simulink model "greenhouse_simulink_part3_pid"  (R2023b)
settings: Solver=VariableStepAuto  StartTime=0.0  StopTime=60*60*24  RelTol=1e-3
undefined symbols (not defined in the file or in its folder): Ca, km1_m2, km1e, km2e, p, t0, thermal_pump, Ts
libraries: slpidlib x2
settings Model: Creator=bianc  LastModifiedBy=bianc
settings OptimizationCC: ReuseModelBlockBuffer=off

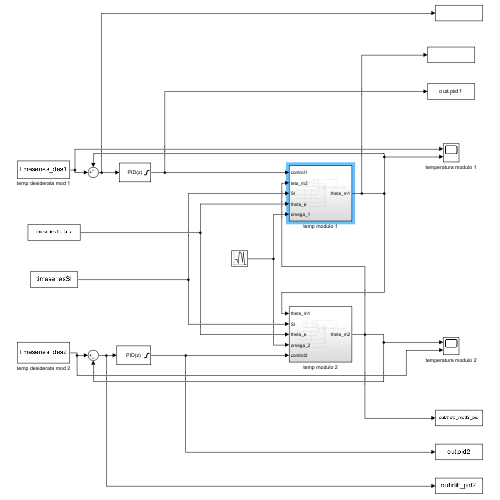
[thumbnail: Simulink's stored preview of the top-level diagram]
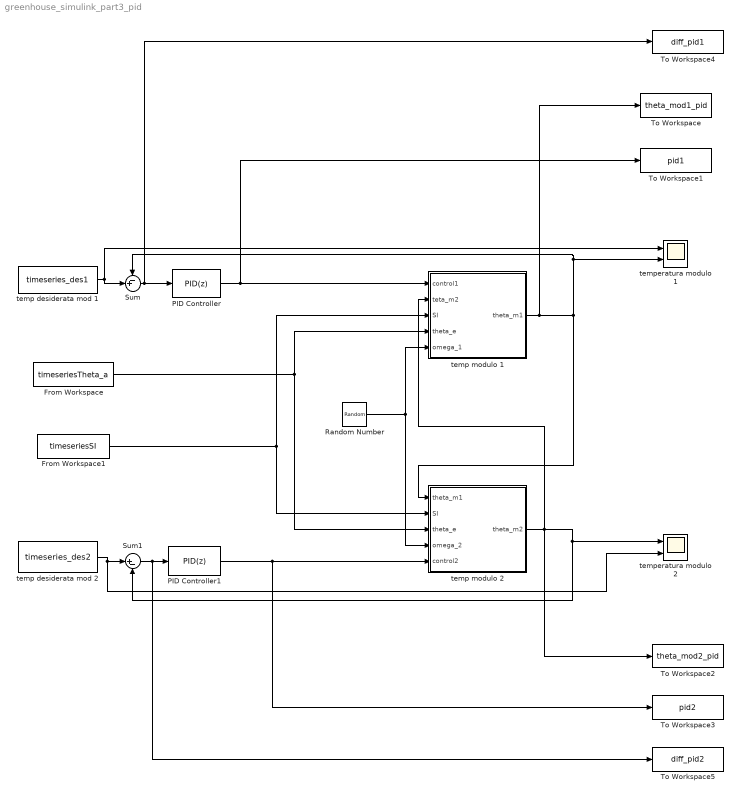
== system greenhouse_simulink_part3_pid ==
  From Workspace : FromWorkspace  VariableName=timeseriesTheta_a
  From Workspace1 : FromWorkspace  VariableName=timeseriesSI
  PID Controller : slpidlib/PID Controller  Controller=PID  Form=Parallel  TimeDomain=Discrete-time  UseExternalTs=off  SampleTime=-1  IntegratorMethod=Forward Euler  FilterMethod=Forward Euler  ControllerParametersSource=internal  P=2076.70497666852  I=18.026617059555  UseKiTs=off  D=-1481.00843350033  N=1.40222359960523  UseFilter=on  TunerSelectOption=Transfer Function Based (PID Tuner App)  InitialConditionSource=internal  InitialConditionForIntegrator=0  InitialConditionForFilter=0  DifferentiatorICPrevScaledInput=0  ExternalReset=none  TrackingMode=off  Kt=1  LimitOutput=on  SatLimitsSource=internal  UpperSaturationLimit=thermal_pump  LowerSaturationLimit=-thermal_pump  LinearizeAsGain=off  AntiWindupMode=none  Kb=1  LimitIntegrator=off  UpperIntegratorSaturationLimit=inf  LowerIntegratorSaturationLimit=-inf  POutMin=[]  POutMax=[]  IOutMin=[]  IOutMax=[]  DOutMin=[]  DOutMax=[]  NOutMin=[]  NOutMax=[]  SumOutMin=[]  SumOutMax=[]  SaturationOutMin=[]  SaturationOutMax=[]  PParamMin=[]  PParamMax=[]  IParamMin=[]  IParamMax=[]  DParamMin=[]  DParamMax=[]  NParamMin=[]  NParamMax=[]  KbParamMin=[]  KbParamMax=[]  KtParamMin=[]  KtParamMax=[]  KbOutMin=[]  KbOutMax=[]  KtOutMin=[]  KtOutMax=[]  IntegratorOutMin=[]  IntegratorOutMax=[]  FilterOutMin=[]  FilterOutMax=[]  SumI1OutMin=[]  SumI1OutMax=[]  SumI2OutMin=[]  SumI2OutMax=[]  SumI3OutMin=[]  SumI3OutMax=[]  SumI4OutMin=[]  SumI4OutMax=[]  SumDOutMin=[]  SumDOutMax=[]  DifferentiatorOutMin=[]  DifferentiatorOutMax=[]  FilterDiffOutCoefMin=[]  FilterDiffOutCoefMax=[]  ReciprocalOutMin=[]  ReciprocalOutMax=[]  SumDenOutMin=[]  SumDenOutMax=[]  SumNumOutMin=[]  SumNumOutMax=[]  DivideOutMin=[]  DivideOutMax=[]  UdiffTsProdOutMin=[]  UdiffTsProdOutMax=[]  NTsProdOutMin=[]  NTsProdOutMax=[]  UintegralTsProdOutMin=[]  UintegralTsProdOutMax=[]  UngainTsProdOutMin=[]  UngainTsProdOutMax=[]  ClampingZeroOutDataTypeStr=Inherit: Inherit via back propagation  ClampingZeroOutMin=[]  ClampingZeroOutMax=[]  FilterDenConstantOutDataTypeStr=Inherit: Inherit via back propagation  FilterDenConstantOutMin=[]  FilterDenConstantOutMax=[]  PCopyOutDataTypeStr=Inherit: Inherit via back propagation  PCopyOutMin=[]  PCopyOutMax=[]  NCopyOutDataTypeStr=Inherit: Inherit via back propagation  NCopyOutMin=[]  NCopyOutMax=[]  IntegratorContinuousStateAttributes=''  IntegratorStateMustResolveToSignalObject=off  IntegratorRTWStateStorageClass=Auto  FilterContinuousStateAttributes=''  FilterStateMustResolveToSignalObject=off  FilterRTWStateStorageClass=Auto  ParallelPVariant=InternalParameters  IdealPVariant=Disabled  IVariant=InternalParameters  DVariant=InternalParameters  IntegratorVariant=Discrete  SatVariant=Enabled  AWVariant=Passthrough  PCopyVariant=Disabled  TRVariant=Disabled  FdbkBlocksVariant=Forward  IdealPFdbkVariant=Disabled  SatFdbkVariant=Disabled  DerivativeFilterVariant=ForwardEulerFilter  NVariant=InternalParameters  NCopyVariant=Disabled  FilterICVariant=InternalICsFilter  IntegratorICVariant=InternalICs  ExternalResetVariant=Disabled  TRSumVariant=Passthrough  SumFdbkVariant=Disabled  SumVariant=Sum_PID  TsampFilterVariant=InternalTs  TsampNgainVariant=Passthrough  TsampIntegralVariant=Disabled_SignalSpec  ExternalSaturationOutDataTypeStr=Inherit: Same as second input
  PID Controller1 : slpidlib/PID Controller  Controller=PID  Form=Parallel  TimeDomain=Discrete-time  UseExternalTs=off  SampleTime=-1  IntegratorMethod=Forward Euler  FilterMethod=Forward Euler  ControllerParametersSource=internal  P=1441.99993550306  I=12.4397713752663  UseKiTs=off  D=-14564.9348598741  N=0.0990049011118977  UseFilter=on  TunerSelectOption=Transfer Function Based (PID Tuner App)  InitialConditionSource=internal  InitialConditionForIntegrator=0  InitialConditionForFilter=0  DifferentiatorICPrevScaledInput=0  ExternalReset=none  TrackingMode=off  Kt=1  LimitOutput=on  SatLimitsSource=internal  UpperSaturationLimit=thermal_pump  LowerSaturationLimit=-thermal_pump  LinearizeAsGain=off  AntiWindupMode=none  Kb=1  LimitIntegrator=off  UpperIntegratorSaturationLimit=inf  LowerIntegratorSaturationLimit=-inf  POutMin=[]  POutMax=[]  IOutMin=[]  IOutMax=[]  DOutMin=[]  DOutMax=[]  NOutMin=[]  NOutMax=[]  SumOutMin=[]  SumOutMax=[]  SaturationOutMin=[]  SaturationOutMax=[]  PParamMin=[]  PParamMax=[]  IParamMin=[]  IParamMax=[]  DParamMin=[]  DParamMax=[]  NParamMin=[]  NParamMax=[]  KbParamMin=[]  KbParamMax=[]  KtParamMin=[]  KtParamMax=[]  KbOutMin=[]  KbOutMax=[]  KtOutMin=[]  KtOutMax=[]  IntegratorOutMin=[]  IntegratorOutMax=[]  FilterOutMin=[]  FilterOutMax=[]  SumI1OutMin=[]  SumI1OutMax=[]  SumI2OutMin=[]  SumI2OutMax=[]  SumI3OutMin=[]  SumI3OutMax=[]  SumI4OutMin=[]  SumI4OutMax=[]  SumDOutMin=[]  SumDOutMax=[]  DifferentiatorOutMin=[]  DifferentiatorOutMax=[]  FilterDiffOutCoefMin=[]  FilterDiffOutCoefMax=[]  ReciprocalOutMin=[]  ReciprocalOutMax=[]  SumDenOutMin=[]  SumDenOutMax=[]  SumNumOutMin=[]  SumNumOutMax=[]  DivideOutMin=[]  DivideOutMax=[]  UdiffTsProdOutMin=[]  UdiffTsProdOutMax=[]  NTsProdOutMin=[]  NTsProdOutMax=[]  UintegralTsProdOutMin=[]  UintegralTsProdOutMax=[]  UngainTsProdOutMin=[]  UngainTsProdOutMax=[]  ClampingZeroOutDataTypeStr=Inherit: Inherit via back propagation  ClampingZeroOutMin=[]  ClampingZeroOutMax=[]  FilterDenConstantOutDataTypeStr=Inherit: Inherit via back propagation  FilterDenConstantOutMin=[]  FilterDenConstantOutMax=[]  PCopyOutDataTypeStr=Inherit: Inherit via back propagation  PCopyOutMin=[]  PCopyOutMax=[]  NCopyOutDataTypeStr=Inherit: Inherit via back propagation  NCopyOutMin=[]  NCopyOutMax=[]  IntegratorContinuousStateAttributes=''  IntegratorStateMustResolveToSignalObject=off  IntegratorRTWStateStorageClass=Auto  FilterContinuousStateAttributes=''  FilterStateMustResolveToSignalObject=off  FilterRTWStateStorageClass=Auto  ParallelPVariant=InternalParameters  IdealPVariant=Disabled  IVariant=InternalParameters  DVariant=InternalParameters  IntegratorVariant=Discrete  SatVariant=Enabled  AWVariant=Passthrough  PCopyVariant=Disabled  TRVariant=Disabled  FdbkBlocksVariant=Forward  IdealPFdbkVariant=Disabled  SatFdbkVariant=Disabled  DerivativeFilterVariant=ForwardEulerFilter  NVariant=InternalParameters  NCopyVariant=Disabled  FilterICVariant=InternalICsFilter  IntegratorICVariant=InternalICs  ExternalResetVariant=Disabled  TRSumVariant=Passthrough  SumFdbkVariant=Disabled  SumVariant=Sum_PID  TsampFilterVariant=InternalTs  TsampNgainVariant=Passthrough  TsampIntegralVariant=Disabled_SignalSpec  ExternalSaturationOutDataTypeStr=Inherit: Same as second input
  Random Number : RandomNumber  SampleTime=1
  Sum : Sum  Inputs=-+|
  Sum1 : Sum  Inputs=|+-
  To Workspace : ToWorkspace  VariableName=theta_mod1_pid  SampleTime=-1
  To Workspace1 : ToWorkspace  VariableName=pid1  SampleTime=-1
  To Workspace2 : ToWorkspace  VariableName=theta_mod2_pid  SampleTime=-1
  To Workspace3 : ToWorkspace  VariableName=pid2  SampleTime=-1
  To Workspace4 : ToWorkspace  VariableName=diff_pid1  SampleTime=-1
  To Workspace5 : ToWorkspace  VariableName=diff_pid2  SampleTime=-1
  temp desiderata mod 1 : FromWorkspace  VariableName=timeseries_des1
  temp desiderata mod 2 : FromWorkspace  VariableName=timeseries_des2
  temp modulo 1 : Subsystem
  temp modulo 2 : Subsystem
  temperatura modulo 1 : Scope  NumInputPorts=2
  temperatura modulo 2 : Scope  NumInputPorts=2
  wires:
  From Workspace1/1 -> temp modulo 1/3(SI), temp modulo 2/2(SI)
  From Workspace/1 -> temp modulo 1/4(theta_e), temp modulo 2/3(theta_e)
  Random Number/1 -> temp modulo 1/5(omega_1), temp modulo 2/4(omega_2)
  temp modulo 2/1(theta_m2) -> temp modulo 1/2(teta_m2), To Workspace2/1, temperatura modulo 2/1, Sum1/2
  temp desiderata mod 1/1 -> Sum/2, temperatura modulo 1/1
  temp modulo 1/1(theta_m1) -> To Workspace/1, Sum/1, temperatura modulo 1/2, temp modulo 2/1(theta_m1)
  temp desiderata mod 2/1 -> temperatura modulo 2/2, Sum1/1
  Sum1/1 -> To Workspace5/1, PID Controller1/1
  PID Controller1/1 -> To Workspace3/1, temp modulo 2/5(control2)
  Sum/1 -> To Workspace4/1, PID Controller/1
  PID Controller/1 -> temp modulo 1/1(control1), To Workspace1/1

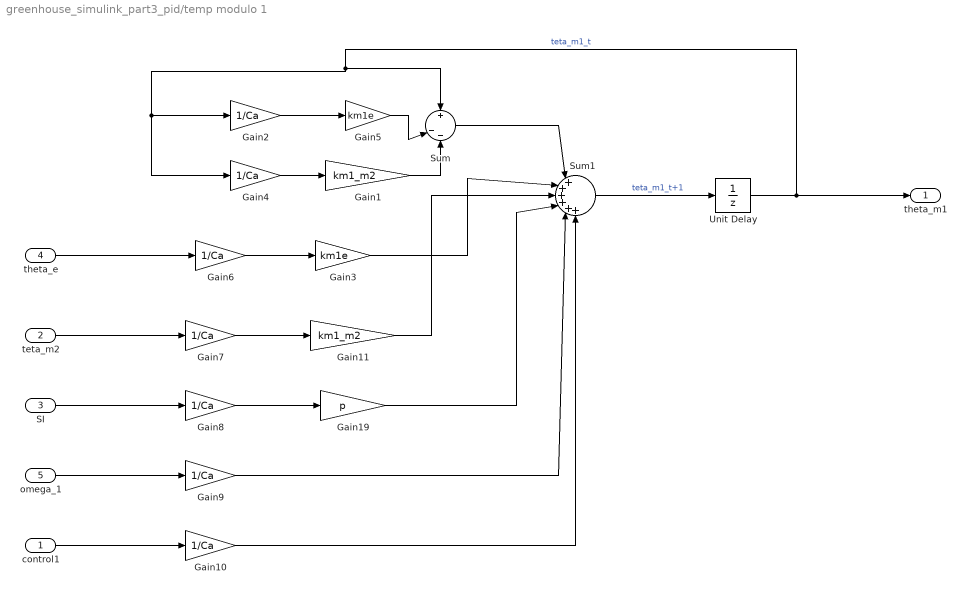
== system greenhouse_simulink_part3_pid/temp modulo 1 ==
  control1 : Inport
  teta_m2 : Inport  Port=2
  SI : Inport  Port=3
  theta_e : Inport  Port=4
  omega_1 : Inport  Port=5
  Gain1 : Gain  Gain=km1_m2
  Gain{2,4,6..10} (7 alike) : Gain  Gain=1/Ca
  Gain11 : Gain  Gain=km1_m2
  Gain19 : Gain  Gain=p
  Gain3 : Gain  Gain=km1e
  Gain5 : Gain  Gain=km1e
  Sum : Sum  Inputs=+|--
  Sum1 : Sum  Inputs=|++++++
  Unit Delay : UnitDelay  InitialCondition=t0  SampleTime=Ts  HasFrameUpgradeWarning=on
  theta_m1 : Outport
  wires:
  Unit Delay/1 -> Sum/1, Gain4/1, Gain2/1, theta_m1/1  "teta_m1_t"
  control1/1 -> Gain10/1
  Sum/1 -> Sum1/1
  teta_m2/1 -> Gain7/1
  omega_1/1 -> Gain9/1
  Gain3/1 -> Sum1/2
  Sum1/1 -> Unit Delay/1  "teta_m1_t+1"
  Gain11/1 -> Sum1/3
  Gain19/1 -> Sum1/4
  SI/1 -> Gain8/1
  theta_e/1 -> Gain6/1
  Gain2/1 -> Gain5/1
  Gain4/1 -> Gain1/1
  Gain6/1 -> Gain3/1
  Gain7/1 -> Gain11/1
  Gain8/1 -> Gain19/1
  Gain9/1 -> Sum1/5
  Gain10/1 -> Sum1/6
  Gain1/1 -> Sum/3
  Gain5/1 -> Sum/2

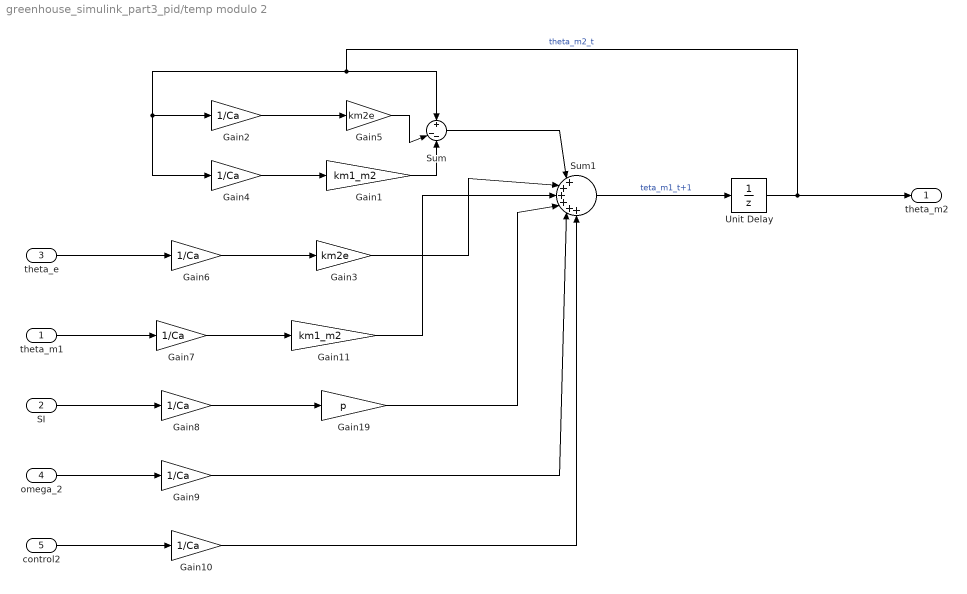
== system greenhouse_simulink_part3_pid/temp modulo 2 ==
  theta_m1 : Inport
  SI : Inport  Port=2
  theta_e : Inport  Port=3
  omega_2 : Inport  Port=4
  control2 : Inport  Port=5
  Gain1 : Gain  Gain=km1_m2
  Gain{2,4,6..10} (7 alike) : Gain  Gain=1/Ca
  Gain11 : Gain  Gain=km1_m2
  Gain19 : Gain  Gain=p
  Gain3 : Gain  Gain=km2e
  Gain5 : Gain  Gain=km2e
  Sum : Sum  Inputs=+|--
  Sum1 : Sum  Inputs=|++++++
  Unit Delay : UnitDelay  InitialCondition=t0  SampleTime=Ts  HasFrameUpgradeWarning=on
  theta_m2 : Outport
  wires:
  Unit Delay/1 -> Sum/1, Gain4/1, Gain2/1, theta_m2/1  "theta_m2_t"
  control2/1 -> Gain10/1
  Sum/1 -> Sum1/1
  theta_m1/1 -> Gain7/1
  omega_2/1 -> Gain9/1
  Gain3/1 -> Sum1/2
  Gain11/1 -> Sum1/3
  Gain19/1 -> Sum1/4
  SI/1 -> Gain8/1
  theta_e/1 -> Gain6/1
  Gain2/1 -> Gain5/1
  Gain4/1 -> Gain1/1
  Gain6/1 -> Gain3/1
  Gain7/1 -> Gain11/1
  Gain8/1 -> Gain19/1
  Gain9/1 -> Sum1/5
  Gain10/1 -> Sum1/6
  Sum1/1 -> Unit Delay/1  "teta_m1_t+1"
  Gain5/1 -> Sum/2
  Gain1/1 -> Sum/3
